simulink model "sys3Tanks_v3"  (Simulink 8.5)
settings: Solver=ode4  StartTime=0  StopTime=54.3  FixedStep=.0005  RelTol=1e-3
values from neighbouring files (symbols this model uses):
  A = [-a, a, 0; a, -a-b, b; 0, b, -b-c]    [tanques.m]
  Ac = A - B*K + L*C    [tanques.m]
  az1 = .511    (= 0.511)    [tanques.m]
  az2 = .528    (= 0.528)    [tanques.m]
  az3 = .731    (= 0.731)    [tanques.m]
  B = [1/S; 0; 0]    [tanques.m]
  Bc = -L    [tanques.m]
  C = [0 0 1]    [tanques.m]
  Cc = K    [tanques.m]
  D = 0    [tanques.m]
  Dc = 0    [tanques.m]
  g = 9.81    [tanques.m]
  h1e = .6    (= 0.6)    [tanques.m]
  h2e = .5    (= 0.5)    [tanques.m]
  h3e = .406    (= 0.406)    [tanques.m]
  K = acker(A, B, pk)    [tanques.m]
  Kr = -1/((C/(A-B*K))*B)    [tanques.m]
  L = acker(A', -C', pl)'    [tanques.m]
  Q1e = .358e-4    (= 3.58e-05)    [tanques.m]
  Q2e = .674e-4    (= 6.74e-05)    [tanques.m]
  S = .0171    (= 0.0171)    [tanques.m]
  S1 = 5e-5    (= 5e-05)    [tanques.m]
  S2 = 5e-5    (= 5e-05)    [tanques.m]
  S3 = 5e-5    (= 5e-05)    [tanques.m]
settings Model: Creator=Victor  LastModifiedBy=joseg
settings DataIOCC: LimitDataPoints=off
settings DebuggingCC: SolverPrmCheckMsg=warning  FcnCallInpInsideContextMsg=UseLocalSettings

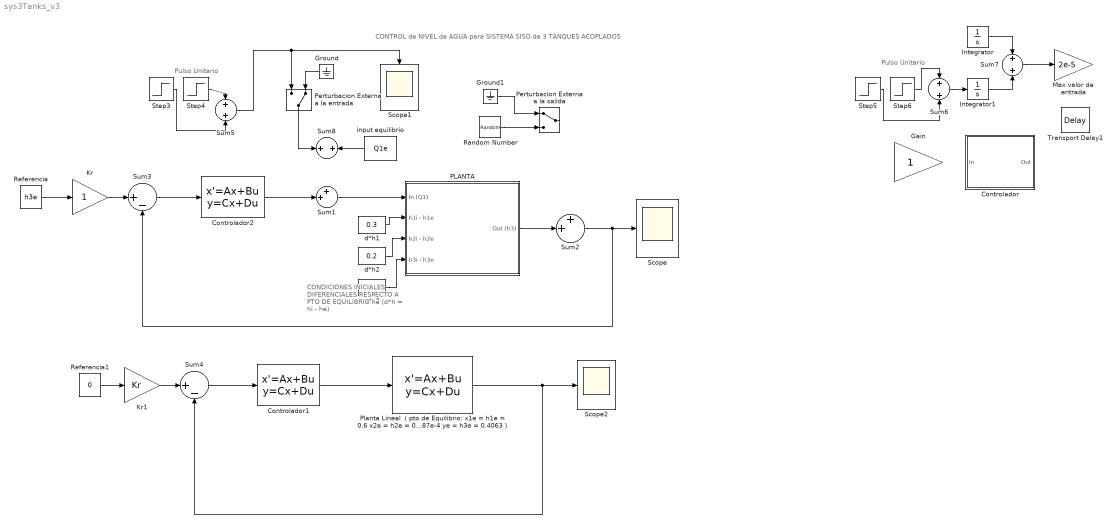
== system sys3Tanks_v3 ==
  note: CONTROL de NIVEL de AGUA para SISTEMA SISO de 3 TANQUES ACOPLADOS
  note: CONDICIONES INICIALES
      | DIFERENCIALES
      | RESPECTO A PTO
      | DE EQUILIBRIO he
      | (d*h = hi - he)
  note: Pulso Unitario
  note: Pulso Unitario
  " input equilibrio" : Constant  Value=Q1e
  Controlador : Subsystem  TreatAsAtomicUnit=on
  Controlador1 : StateSpace  A=Ac  B=Bc  C=Cc  D=Dc  X0=[0;0;0]
  Controlador2 : StateSpace  A=Ac  B=Bc  C=Cc  D=Dc  X0=[0;0;0]
  Gain : Gain
  Ground : Ground
  Ground1 : Ground
  Integrator : Integrator
  Integrator1 : Integrator
  Kr : Gain
  Kr1 : Gain  Gain=Kr
  Max valor de entrada : Gain  Gain=2e-5
  PLANTA : Subsystem  TreatAsAtomicUnit=on
  Perturbacion Externa a la entrada : ManualSwitch  CurrentSetting=0
  Perturbacion Externa a la salida : ManualSwitch
  Planta Lineal  ( pto de Equilibrio: x1e = h1e = 0.6 x2e = h2e = 0.5 x3e = h3e = 0.4063 ue = Q1e = 0.35787e-4 ye = h3e = 0.4063 ) : StateSpace  A=A  B=B  C=C  D=D  X0=[1.2; 0.9; 0.1]
  Random Number : RandomNumber  Variance=1e-6
  Referencia : Constant  Value=h3e
  Referencia1 : Constant  Value=0
  Scope : Scope
      settings: TimeRange=14.3  YMin=0.5  YMax=0.775
  Scope1 : Scope
      settings: TimeRange=300  YMin=0.38  YMax=0.47
  Scope2 : Scope
      settings: TimeRange=4.5  YMin=0.01425  YMax=0.01975  SaveName=ScopeData2
  Step3 : Step  Before=-0.5  After=0.5  SampleTime=0
  Step4 : Step  Time=1.5  Before=0.5  After=-0.5  SampleTime=0
  Step5 : Step  Time=2  Before=0.5  After=-0.5  SampleTime=0
  Step6 : Step  Time=2.5  Before=-0.5  After=0.5  SampleTime=0
  Sum1 : Sum  Inputs=++|
  Sum2 : Sum  Inputs=++|
  Sum3 : Sum  Inputs=|+-
  Sum4 : Sum  Inputs=|+-
  Sum{5..8} (4 alike) : Sum  Inputs=+|+
  Transport Delay1 : TransportDelay  DelayTime=3
  d*h1 : Constant  Value=0.3
  d*h2 : Constant  Value=0.2
  d*h3 : Constant  Value=0.1
  wires:
  Sum1/1 -> PLANTA/1(In (Q1))
  Sum2/1 -> Scope/1, Sum3/2
  PLANTA/1(Out (h3)) -> Sum2/2
  Ground/1 -> Perturbacion Externa a la entrada/2
  Ground1/1 -> Perturbacion Externa a la salida/1
  Step4/1 -> Sum5/1
  Step3/1 -> Sum5/2
  Step6/1 -> Sum6/1
  Step5/1 -> Sum6/2
  Sum6/1 -> Integrator1/1
  Integrator/1 -> Sum7/1
  Integrator1/1 -> Sum7/2
  Sum5/1 -> Scope1/1, Perturbacion Externa a la entrada/1
  Sum7/1 -> Max valor de entrada/1
  Random Number/1 -> Perturbacion Externa a la salida/2
  Planta Lineal  ( pto de Equilibrio: x1e = h1e = 0.6 x2e = h2e = 0.5 x3e = h3e = 0.4063 ue = Q1e = 0.35787e-4 ye = h3e = 0.4063 )/1 -> Sum4/2, Scope2/1
  Sum4/1 -> Controlador1/1
  Referencia1/1 -> Kr1/1
  " input equilibrio"/1 -> Sum8/2
  Kr1/1 -> Sum4/1
  Controlador1/1 -> Planta Lineal  ( pto de Equilibrio: x1e = h1e = 0.6 x2e = h2e = 0.5 x3e = h3e = 0.4063 ue = Q1e = 0.35787e-4 ye = h3e = 0.4063 )/1
  Sum3/1 -> Controlador2/1
  Controlador2/1 -> Sum1/2
  d*h1/1 -> PLANTA/2(h1i - h1e)
  d*h2/1 -> PLANTA/3(h2i - h2e)
  d*h3/1 -> PLANTA/4(h3i - h3e)
  Kr/1 -> Sum3/1
  Referencia/1 -> Kr/1
  Perturbacion Externa a la entrada/1 -> Sum8/1

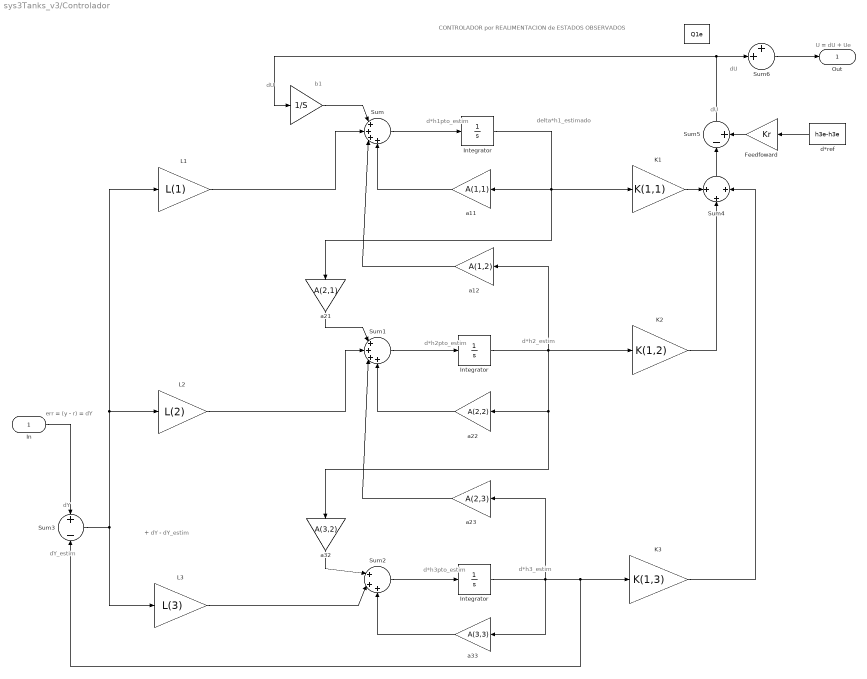
== system sys3Tanks_v3/Controlador ==
  note: dY_estim
  note: d*h1pto_estim
  note: delta*h1_estimado
  note: d*h2pto_estim
  note: d*h2_estim
  note: d*h3pto_estim
  note: d*h3_estim
  note: dU
  note: CONTROLADOR por REALIMENTACION de ESTADOS OBSERVADOS
  note: err = (y - r) = dY
  note: dY
  note: dU
  note: U = dU + Ue
  note: dU
  note: b1
  note: + dY - dY_estim
  In : Inport
  " " : Constant  Value=Q1e
  "   " : Gain  Gain=1/S
  " Integrator " : Integrator
  Feedfoward : Gain  Gain=Kr
  Integrator : Integrator
  "Integrator  " : Integrator
  K1 : Gain  Gain=K(1,1)
  K2 : Gain  Gain=K(1,2)
  K3 : Gain  Gain=K(1,3)
  L1 : Gain  Gain=L(1)
  L2 : Gain  Gain=L(2)
  L3 : Gain  Gain=L(3)
  Sum : Sum  Inputs=|++++
  Sum1 : Sum  Inputs=|++++
  Sum2 : Sum  Inputs=|+++
  Sum3 : Sum  Inputs=+|-
  Sum4 : Sum  Inputs=+|+|+
  Sum5 : Sum  Inputs=|-+
  Sum6 : Sum  Inputs=++|
  a11 : Gain  Gain=A(1,1)
  a12 : Gain  Gain=A(1,2)
  a21 : Gain  Gain=A(2,1)
  a22 : Gain  Gain=A(2,2)
  a23 : Gain  Gain=A(2,3)
  a32 : Gain  Gain=A(3,2)
  a33 : Gain  Gain=A(3,3)
  "d*ref  " : Constant  Value=h3e-h3e
  Out : Outport
  wires:
  Integrator/1 -> a11/1, K1/1, a21/1
  Sum/1 -> Integrator/1
  "   "/1 -> Sum/1
  "Integrator  "/1 -> a12/1, a22/1, a32/1, K2/1
  Sum1/1 -> "Integrator  "/1
  a21/1 -> Sum1/1
  " Integrator "/1 -> a33/1, a23/1, K3/1, Sum3/2
  Sum2/1 -> " Integrator "/1
  a32/1 -> Sum2/1
  Sum3/1 -> L2/1, L1/1, L3/1
  K1/1 -> Sum4/1
  K3/1 -> Sum4/3
  K2/1 -> Sum4/2
  Sum5/1 -> "   "/1, Sum6/2
  Feedfoward/1 -> Sum5/2
  "d*ref  "/1 -> Feedfoward/1
  Sum6/1 -> Out/1
  L3/1 -> Sum2/2
  a33/1 -> Sum2/3
  L2/1 -> Sum1/2
  a23/1 -> Sum1/3
  a22/1 -> Sum1/4
  L1/1 -> Sum/2
  a11/1 -> Sum/4
  a12/1 -> Sum/3
  Sum4/1 -> Sum5/1
  In/1 -> Sum3/1

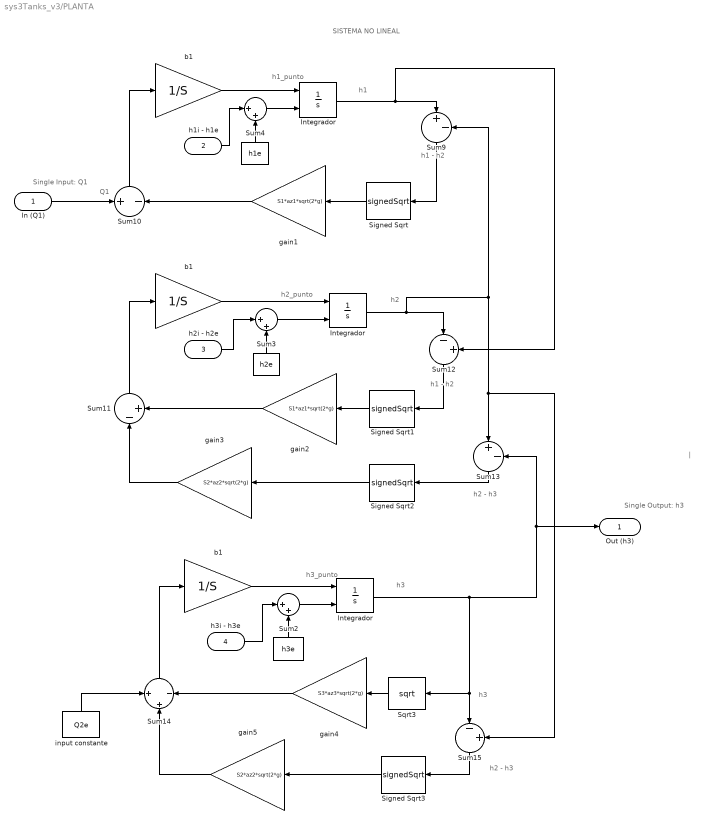
== system sys3Tanks_v3/PLANTA ==
  note: |
  note: Q1
  note: h2 - h3
  note: h1 - h2
  note: h1 - h2
  note: h2 - h3
  note: h3
  note: h3
  note: h3_punto
  note: h2
  note: h2_punto
  note: h1_punto
  note: h1
  note: Single Input: Q1
  note: Single Output: h3
  note: SISTEMA NO LINEAL
  In (Q1) : Inport
  h1i - h1e : Inport  Port=2
  h2i - h2e : Inport  Port=3
  h3i - h3e : Inport  Port=4
  " " : Constant  Value=h1e
  "   " : Constant  Value=h2e
  "     " : Constant  Value=h3e
  " Integrador  " : Integrator  InitialConditionSource=external  InitialCondition=0.406  LimitOutput=on  UpperSaturationLimit=1e2  LowerSaturationLimit=0  AbsoluteTolerance=1
  " b1 " : Gain  Gain=1/S
  " input constante" : Constant  Value=Q2e
  Integrador : Integrator  InitialConditionSource=external  InitialCondition=0.5
  "Integrador " : Integrator  InitialConditionSource=external  InitialCondition=0.6
  Signed Sqrt{,1..3} (4 alike) : Sqrt  Operator=signedSqrt  SaturateOnIntegerOverflow=on
  Sqrt3 : Sqrt  OutputSignalType=real  SaturateOnIntegerOverflow=on
  Sum10 : Sum  Inputs=+|-
  Sum11 : Sum  Inputs=|-+
  Sum12 : Sum  Inputs=|-+
  Sum13 : Sum  Inputs=|+-
  Sum14 : Sum  Inputs=+|+|-
  Sum15 : Sum  Inputs=|-+
  Sum2 : Sum  Inputs=|++
  Sum3 : Sum  Inputs=|++
  Sum4 : Sum  Inputs=|++
  Sum9 : Sum  Inputs=|+-
  b1 : Gain  Gain=1/S
  "b1   " : Gain  Gain=1/S
  gain1 : Gain  Gain=S1*az1*sqrt(2*g)
  gain2 : Gain  Gain=S1*az1*sqrt(2*g)
  gain3 : Gain  Gain=S2*az2*sqrt(2*g)
  gain4 : Gain  Gain=S3*az3*sqrt(2*g)
  gain5 : Gain  Gain=S2*az2*sqrt(2*g)
  Out (h3) : Outport
  wires:
  "Integrador "/1 -> Sum12/2, Sum9/1
  b1/1 -> "Integrador "/1
  Sum10/1 -> b1/1
  Integrador/1 -> Sum12/1, Sum9/2, Sum13/1, Sum15/2
  "b1   "/1 -> Integrador/1
  Sum11/1 -> "b1   "/1
  " Integrador  "/1 -> Sum15/1, Sqrt3/1, Sum13/2, Out (h3)/1
  Sqrt3/1 -> gain4/1
  " b1 "/1 -> " Integrador  "/1
  Sum14/1 -> " b1 "/1
  gain4/1 -> Sum14/3
  Sum9/1 -> Signed Sqrt/1
  Signed Sqrt/1 -> gain1/1
  gain2/1 -> Sum11/2
  Signed Sqrt1/1 -> gain2/1
  Sum12/1 -> Signed Sqrt1/1
  Signed Sqrt2/1 -> gain3/1
  Sum13/1 -> Signed Sqrt2/1
  gain3/1 -> Sum11/1
  Sum15/1 -> Signed Sqrt3/1
  Signed Sqrt3/1 -> gain5/1
  gain5/1 -> Sum14/2
  " input constante"/1 -> Sum14/1
  In (Q1)/1 -> Sum10/1
  Sum2/1 -> " Integrador  "/2
  "     "/1 -> Sum2/2
  h3i - h3e/1 -> Sum2/1
  "   "/1 -> Sum3/2
  Sum3/1 -> Integrador/2
  h2i - h2e/1 -> Sum3/1
  " "/1 -> Sum4/2
  h1i - h1e/1 -> Sum4/1
  Sum4/1 -> "Integrador "/2
  gain1/1 -> Sum10/2
